simulink model "ejercicio10seguidor"  (R2013a)
settings: Solver=ode45  StartTime=0.0  StopTime=10.0  RelTol=1e-3
values from neighbouring files (symbols this model uses):
  h = h'    [ejercicio10.m]
  ki = kt(1,3)    [ejercicio10.m]
  kp = kt(1,1:2)    [ejercicio10.m]
undefined symbols (not defined in the file or in its folder): a, b, c
settings Model: Creator=mario  LastModifiedBy=mario

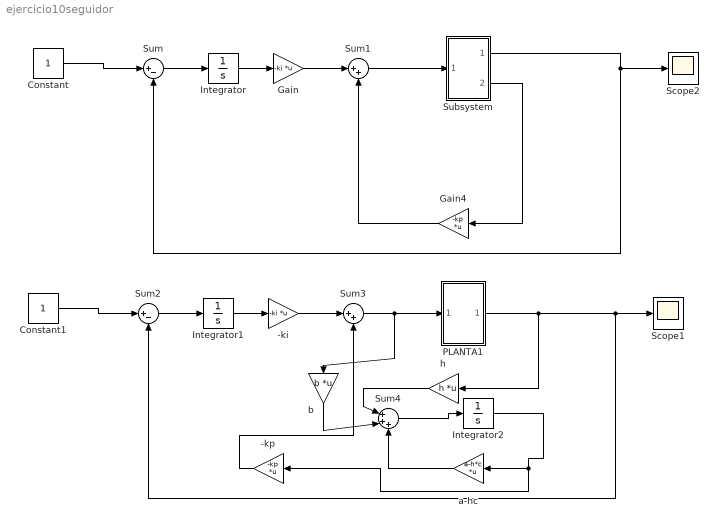
== system ejercicio10seguidor ==
  "-ki " : Gain  Gain=-ki  Multiplication=Matrix(K*u) (u vector)
  -kp : Gain  Gain=-kp  Multiplication=Matrix(K*u) (u vector)
  Constant : Constant
  Constant1 : Constant
  Gain : Gain  Gain=-ki  Multiplication=Matrix(K*u) (u vector)
  Gain4 : Gain  Gain=-kp  Multiplication=Matrix(K*u) (u vector)
  Integrator : Integrator
  Integrator1 : Integrator
  Integrator2 : Integrator
  PLANTA1 : Subsystem
  Scope1 : Scope
  Scope2 : Scope
  Subsystem : Subsystem
  Sum : Sum  Inputs=|+-
  Sum1 : Sum  Inputs=|++
  Sum2 : Sum  Inputs=|+-
  Sum3 : Sum  Inputs=|++
  Sum4 : Sum  Inputs=|+++
  a-hc : Gain  Gain=a-h*c  Multiplication=Matrix(K*u) (u vector)
  b : Gain  Gain=b  Multiplication=Matrix(K*u) (u vector)
  h : Gain  Gain=h  Multiplication=Matrix(K*u) (u vector)
  wires:
  Sum/1 -> Integrator/1
  Integrator/1 -> Gain/1
  Gain/1 -> Sum1/1
  Gain4/1 -> Sum1/2
  Constant/1 -> Sum/1
  Subsystem/1(Out1) -> Scope2/1, Sum/2
  Sum1/1 -> Subsystem/1(In1)
  Subsystem/2(Out2) -> Gain4/1
  Sum2/1 -> Integrator1/1
  Integrator1/1 -> "-ki "/1
  "-ki "/1 -> Sum3/1
  Constant1/1 -> Sum2/1
  PLANTA1/1(Out1) -> h/1, Scope1/1, Sum2/2
  Sum3/1 -> b/1, PLANTA1/1(In1)
  h/1 -> Sum4/1
  b/1 -> Sum4/2
  Sum4/1 -> Integrator2/1
  Integrator2/1 -> -kp/1, a-hc/1
  a-hc/1 -> Sum4/3
  -kp/1 -> Sum3/2

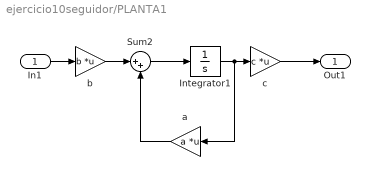
== system ejercicio10seguidor/PLANTA1 ==
  In1 : Inport
  Integrator1 : Integrator
  Sum2 : Sum  Inputs=|++
  a : Gain  Gain=a  Multiplication=Matrix(K*u) (u vector)
  b : Gain  Gain=b  Multiplication=Matrix(K*u) (u vector)
  c : Gain  Gain=c  Multiplication=Matrix(K*u) (u vector)
  Out1 : Outport
  wires:
  Sum2/1 -> Integrator1/1
  c/1 -> Out1/1
  a/1 -> Sum2/2
  b/1 -> Sum2/1
  In1/1 -> b/1
  Integrator1/1 -> c/1, a/1

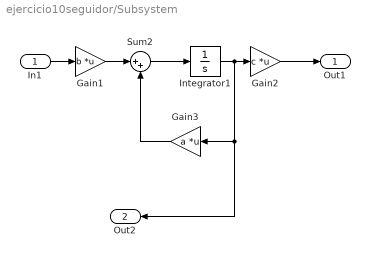
== system ejercicio10seguidor/Subsystem ==
  In1 : Inport
  Gain1 : Gain  Gain=b  Multiplication=Matrix(K*u) (u vector)
  Gain2 : Gain  Gain=c  Multiplication=Matrix(K*u) (u vector)
  Gain3 : Gain  Gain=a  Multiplication=Matrix(K*u) (u vector)
  Integrator1 : Integrator
  Sum2 : Sum  Inputs=|++
  Out1 : Outport
  Out2 : Outport  Port=2
  wires:
  Integrator1/1 -> Out2/1, Gain3/1, Gain2/1
  In1/1 -> Gain1/1
  Gain1/1 -> Sum2/1
  Gain3/1 -> Sum2/2
  Gain2/1 -> Out1/1
  Sum2/1 -> Integrator1/1
